simulink library "SAEJ1939"  (Simulink 7.6)
settings: Solver=ode1  StartTime=0.0  StopTime=Inf  FixedStep=0.001  RelTol=1e-3
PostLoadFcn:
  | , if any(exist('dsrtsu_mdlpostloadfcn', 'file') == [2, 3, 6]), try dsrtsu_mdlpostloadfcn('Execute', bdroot); catch fprintf('Error in PostLoadFcn (dsrtsu_mdlpostloadfcn) for model "%s":\n %s\n', bdroot, lasterr); end, end,
libraries: rtican x15
(part 1 of 2)
settings Model: DSRTSU_INTERNAL_RTI_VER=370  DSRTSU_INTERNAL_RTI_TYPE=rti1401  Creator=ses  LastModifiedBy=ses

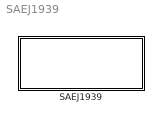
== system SAEJ1939 ==
  SAEJ1939 : Subsystem
